simulink model "auv_reference"  (R2021a)
settings: Solver=VariableStepAuto  StartTime=0.0  StopTime=180.0  RelTol=1e-3
settings Model: Creator=mluser  LastModifiedBy=mluser

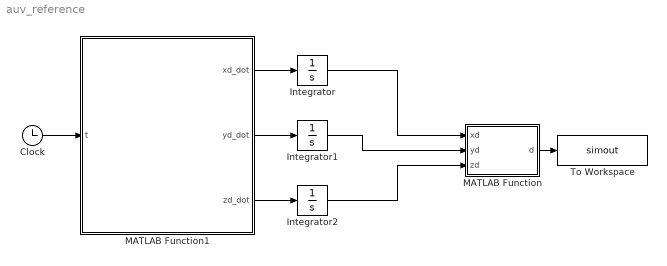
== system auv_reference ==
  Clock : Clock
  Integrator : Integrator
  Integrator1 : Integrator
  Integrator2 : Integrator
  MATLAB Function : MATLAB Function  TreatAsAtomicUnit=on
  MATLAB Function1 : MATLAB Function  TreatAsAtomicUnit=on
  To Workspace : ToWorkspace  VariableName=simout  SaveFormat=Timeseries  SampleTime=-1
  wires:
  Clock/1 -> MATLAB Function1/1(t)
  MATLAB Function1/1(xd_dot) -> Integrator/1
  MATLAB Function1/2(yd_dot) -> Integrator1/1
  MATLAB Function1/3(zd_dot) -> Integrator2/1
  Integrator/1 -> MATLAB Function/1(xd)
  Integrator1/1 -> MATLAB Function/2(yd)
  Integrator2/1 -> MATLAB Function/3(zd)
  MATLAB Function/1(d) -> To Workspace/1

== matlab function auv_reference/MATLAB Function1 ==
  data: xd_dot output; yd_dot output; zd_dot output; t input
function [xd_dot , yd_dot, zd_dot] = fcn(t)
    
    if(t<=90)
        uld =  1.5;
        theta_ld = 0;
        psi_ld = 0;
    else
        uld = 1.5;
        theta_ld = -10;
        psi_ld = 0.06;
    end
    xd_dot = uld*cos(theta_ld)*cos(psi_ld);
    yd_dot = uld*cos(theta_ld)*sin(psi_ld);
    zd_dot = -uld*sin(theta_ld);
  
end

== matlab function auv_reference/MATLAB Function ==
  data: xd input; yd input; zd input; d output
function d = fcn(xd,yd,zd)
    d = [xd yd zd]';
    

end
